simulink model "ExampleFigures"  (R2021b)
settings: Solver=VariableStepAuto  StartTime=0.0  StopTime=10.0  RelTol=1e-3
libraries: Lib_EMTAT x4
settings Model: Creator=sbianco1  LastModifiedBy=sbianco1
settings DebuggingCC: UnconnectedInputMsg=none  UnconnectedOutputMsg=none  UnconnectedLineMsg=none
settings ModelReferenceCC: EnableRefExpFcnMdlSchedulingChecks=off
settings RTWCC: DLArmComputeVersion=20.02.1

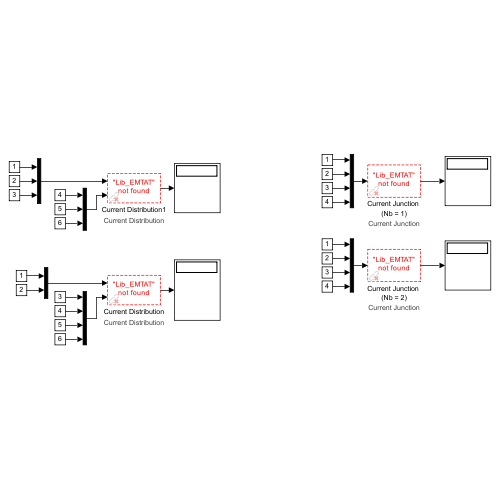
[thumbnail: Simulink's stored preview of the top-level diagram]
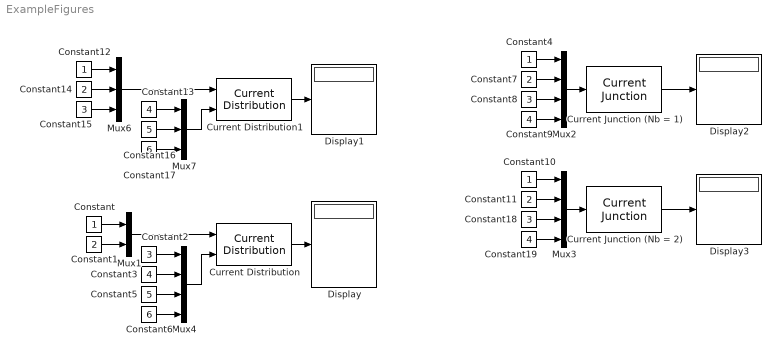
== system ExampleFigures ==
  Constant{,4,10,12} (4 alike) : Constant
  Constant{1,7,11,14} (4 alike) : Constant  Value=2
  Constant{3,9,13,19} (4 alike) : Constant  Value=4
  Constant{2,8,15,18} (4 alike) : Constant  Value=3
  Constant16 : Constant  Value=5
  Constant17 : Constant  Value=6
  Constant5 : Constant  Value=5
  Constant6 : Constant  Value=6
  Current Distribution : Lib_EMTAT/Components/Power Flow/Current Distribution
      settings: AttributesFormatString=Current Distribution  SourceProductName=EMTAT
  Current Distribution1 : Lib_EMTAT/Components/Power Flow/Current Distribution
      settings: AttributesFormatString=Current Distribution  SourceProductName=EMTAT
  Current Junction (Nb = 1) : Lib_EMTAT/Components/Power Flow/Current Junction  Nb=1
      settings: AttributesFormatString=Current Junction  SourceProductName=EMTAT
  Current Junction (Nb = 2) : Lib_EMTAT/Components/Power Flow/Current Junction  Nb=2
      settings: AttributesFormatString=Current Junction  SourceProductName=EMTAT
  Display{,1..3} (4 alike) : Display
  Mux1 : Mux  Inputs=2
  Mux2 : Mux
  Mux3 : Mux
  Mux4 : Mux
  Mux6 : Mux  Inputs=3
  Mux7 : Mux  Inputs=3
  wires:
  Mux1/1 -> Current Distribution/1
  Constant/1 -> Mux1/1
  Constant1/1 -> Mux1/2
  Constant3/1 -> Mux4/2
  Mux4/1 -> Current Distribution/2
  Current Distribution/1 -> Display/1
  Constant5/1 -> Mux4/3
  Constant6/1 -> Mux4/4
  Constant13/1 -> Mux7/1
  Constant14/1 -> Mux6/2
  Constant15/1 -> Mux6/3
  Mux7/1 -> Current Distribution1/2
  Constant12/1 -> Mux6/1
  Constant17/1 -> Mux7/3
  Constant16/1 -> Mux7/2
  Current Distribution1/1 -> Display1/1
  Mux6/1 -> Current Distribution1/1
  Constant2/1 -> Mux4/1
  Current Junction (Nb = 1)/1 -> Display2/1
  Constant4/1 -> Mux2/1
  Constant9/1 -> Mux2/4
  Constant8/1 -> Mux2/3
  Mux2/1 -> Current Junction (Nb = 1)/1
  Constant7/1 -> Mux2/2
  Constant11/1 -> Mux3/2
  Constant18/1 -> Mux3/3
  Constant19/1 -> Mux3/4
  Mux3/1 -> Current Junction (Nb = 2)/1
  Constant10/1 -> Mux3/1
  Current Junction (Nb = 2)/1 -> Display3/1
